simulink model "Third2model"  (R2017b)
settings: Solver=VariableStepAuto  StartTime=0.0  StopTime=10.0  RelTol=1e-3
settings Model: Creator=17863  LastModifiedBy=17863

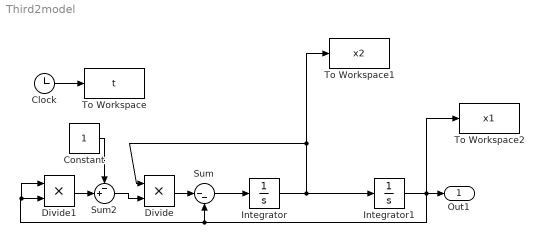
== system Third2model ==
  Clock : Clock
  Constant : Constant
  Divide : Product  Inputs=**
  Divide1 : Product  Inputs=**
  Integrator : Integrator  InitialCondition=1
  Integrator1 : Integrator  InitialCondition=1
  Sum : Sum  Inputs=|--
  Sum2 : Sum  Inputs=-+|
  To Workspace : ToWorkspace  VariableName=t  SampleTime=-1
      settings: Save2DSignal=2-D array (concatenate along first dimension)
  To Workspace1 : ToWorkspace  VariableName=x2  SampleTime=-1
      settings: Save2DSignal=2-D array (concatenate along first dimension)
  To Workspace2 : ToWorkspace  VariableName=x1  SampleTime=-1
      settings: Save2DSignal=2-D array (concatenate along first dimension)
  Out1 : Outport
  wires:
  Clock/1 -> To Workspace/1
  Sum/1 -> Integrator/1
  Integrator/1 -> Integrator1/1, Divide/1, To Workspace1/1
  Integrator1/1 -> Divide1/1, Divide1/2, Sum/2, To Workspace2/1, Out1/1
  Divide/1 -> Sum/1
  Divide1/1 -> Sum2/2
  Constant/1 -> Sum2/1
  Sum2/1 -> Divide/2
